simulink model "polyphaseChannelizer"  (R2023b)
settings: Solver=FixedStepDiscrete  StartTime=0.0  StopTime=0.001  RelTol=1e-3
undefined symbols (not defined in the file): parula
libraries: dspobslib x4, dspmlti4 x4, dspmathops x4, radarlib x1, phasedwavlib x1, commdigbbndfm2 x1, commrandsrc3 x1
settings Model: Creator=krsh  LastModifiedBy=krsh
settings SolverCC: AlgebraicLoopSolver=TrustRegion  AutoInsertRateTranBlk=on
settings DataIOCC: LimitDataPoints=on  SaveOutput=off  SignalLogging=off  SaveTime=off
settings OptimizationCC: ReuseModelBlockBuffer=off  LifeSpan=inf  SimCompilerOptimization=on
settings DebuggingCC: AlgebraicLoopMsg=error  SingleTaskRateTransMsg=error  UnconnectedInputMsg=warning  UnconnectedOutputMsg=warning  UnconnectedLineMsg=warning  AllowSymbolicDim=off  SubsystemReferenceDiagnosticForUnitTest=warning  SFUnexpectedBacktrackingDiag=warning  SFNoUnconditionalDefaultTransitionDiag=warning  SFExecutionAtInitializationDiag=none  ArithmeticOperatorsInVariantConditions=warning
settings ModelReferenceCC: EnableRefExpFcnMdlSchedulingChecks=on
settings SFSimCC: SimUseLocalCustomCode=off  CustomCodeUndefinedFunction=UseInterfaceOnly
settings RTWCC: RTWUseLocalCustomCode=off
settings CodeAppCC: StateflowObjectComments=on
settings GRTTargetCC: TargetLangStandard=C89/C90 (ANSI)
settings ConfigComp: CovMetricSettings=dw  CovSaveCumulativeToWorkspaceVar=on  CovSaveSingleToWorkspaceVar=on  CovExternalEMLEnable=off  CovSFcnEnable=off

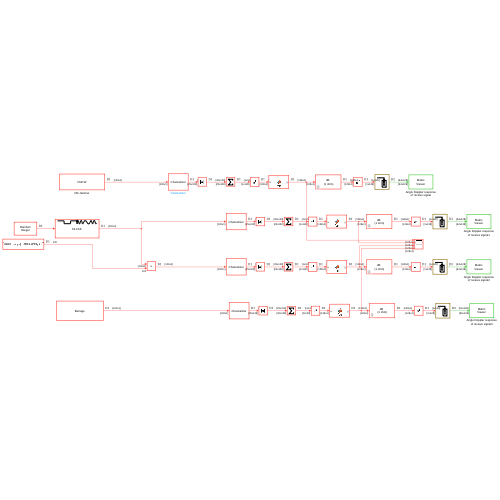
[thumbnail: Simulink's stored preview of the top-level diagram]
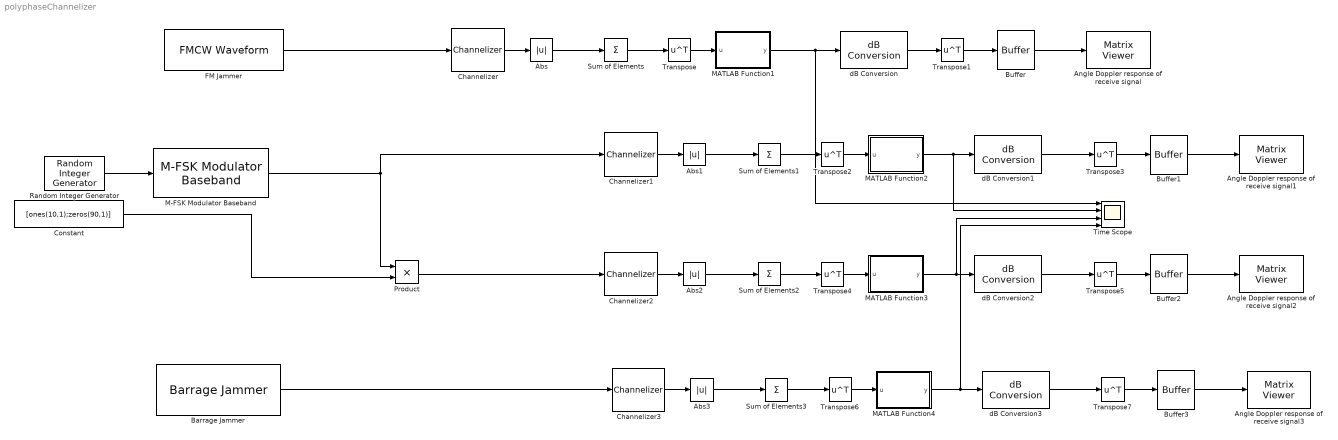
== system polyphaseChannelizer ==
  Abs{,1..3} (4 alike) : Abs  SaturateOnIntegerOverflow=off
  Angle Doppler response of receive signal{,1..3} (4 alike) : dspobslib/Matrix Viewer  ImageParams=off  CMapStr=parula(256)  AxisColorbar=on  AxisParams=off  AxisOrigin=Lower left corner  AxisTickMode=User-defined  XTickRange=[-50e6 50e6]  YTickRange=[0 63]  XLabel=FrequencyBand  YLabel=Sweeps  ZLabel=WaterFallScope  FigPos=[50 360 400 300]  AxisZoom=off
      Angle Doppler response of receive signal settings: YMin=-77.8046  YMax=16.5709
      Angle Doppler response of receive signal1 settings: YMin=-40.3602  YMax=24.0141
      Angle Doppler response of receive signal2 settings: YMin=-34.9744  YMax=8.5209
      Angle Doppler response of receive signal3 settings: YMin=-19.8751  YMax=15.4262
  Barrage Jammer : radarlib/Barrage Jammer  ERP=1  SamplesPerFrameSource=Property  SamplesPerFrame=100  SeedSource=Auto  Seed=0  SimulateUsing=Interpreted execution
  Buffer{,1..3} (4 alike) : Buffer  OutputFrames=off
  Channelizer{,1..3} (4 alike) : dspmlti4/Channelizer  NumFrequencyBands=128  Specification=Number of taps per band and stopband attenuation  DecimationFactor=4  CoefficientsPort=off  NumTapsPerBand=12  StopbandAttenuation=80  LowpassCoefficients=rcosdesign( 0.25, 6, 8, 'sqrt' )  AllowArbitraryInputLength=off  SimulateUsing=Interpreted execution
  Constant : Constant  Value=[ones(10,1);zeros(90,1)]  SampleTime=-1
  FM Jammer : phasedwavlib/FMCW Waveform  SampleRate=100e6  SweepTime=1e-6  SweepBandwidth=30e6  SweepDirection=Triangle  SweepInterval=Symmetric  OutputFormat=Sweeps  NumSamples=100  NumSweeps=1  SimulateUsing=Interpreted execution
  M-FSK Modulator Baseband : commdigbbndfm2/M-FSK Modulator Baseband  M=64  InType=Integer  Enc=Gray  freqSep=100e6/64  phaseType=Continuous  numSamp=100  RateOptions=Enforce single-rate processing  outDataType=double
  MATLAB Function1 : MATLAB Function  TreatAsAtomicUnit=on
  MATLAB Function2 : MATLAB Function  TreatAsAtomicUnit=on
  MATLAB Function3 : MATLAB Function  TreatAsAtomicUnit=on
  MATLAB Function4 : MATLAB Function  TreatAsAtomicUnit=on
  Product : Product
  Random Integer Generator : commrandsrc3/Random Integer Generator  SetSize=64  SeedSource=Auto  Seed=0  SampleTime=1/1e6  SamplesPerFrame=1  OutputDataType=double  SimulateUsing=Interpreted execution
  Sum of Elements{,1..3} (4 alike) : Sum  Inputs=+  CollapseMode=Specified dimension
  Time Scope : Scope  NumInputPorts=4
  Transpose{,1..7} (8 alike) : Math  Operator=transpose
  dB Conversion{,1..3} (4 alike) : dspmathops/dB Conversion  dBtype=dB  intype=Amplitude  R=1  fuzz=off
      settings: LibrarySourceBlock=commutil2/dB Conversion
  wires:
  Random Integer Generator/1 -> M-FSK Modulator Baseband/1
  FM Jammer/1 -> Channelizer/1
  M-FSK Modulator Baseband/1 -> Channelizer1/1, Product/1
  Constant/1 -> Product/2
  Channelizer/1 -> Abs/1
  Abs/1 -> Sum of Elements/1
  Sum of Elements/1 -> Transpose/1
  Transpose/1 -> MATLAB Function1/1(u)
  Transpose1/1 -> Buffer/1
  Buffer/1 -> Angle Doppler response of receive signal/1
  dB Conversion/1 -> Transpose1/1
  dB Conversion1/1 -> Transpose3/1
  Buffer1/1 -> Angle Doppler response of receive signal1/1
  Transpose3/1 -> Buffer1/1
  MATLAB Function2/1(y) -> Time Scope/2, dB Conversion1/1
  Transpose2/1 -> MATLAB Function2/1(u)
  Sum of Elements1/1 -> Transpose2/1
  Abs1/1 -> Sum of Elements1/1
  Channelizer1/1 -> Abs1/1
  Channelizer2/1 -> Abs2/1
  Abs2/1 -> Sum of Elements2/1
  Sum of Elements2/1 -> Transpose4/1
  Transpose4/1 -> MATLAB Function3/1(u)
  MATLAB Function3/1(y) -> Time Scope/3, dB Conversion2/1
  Transpose5/1 -> Buffer2/1
  Buffer2/1 -> Angle Doppler response of receive signal2/1
  dB Conversion2/1 -> Transpose5/1
  Product/1 -> Channelizer2/1
  dB Conversion3/1 -> Transpose7/1
  Buffer3/1 -> Angle Doppler response of receive signal3/1
  Transpose7/1 -> Buffer3/1
  MATLAB Function4/1(y) -> Time Scope/4, dB Conversion3/1
  Transpose6/1 -> MATLAB Function4/1(u)
  Sum of Elements3/1 -> Transpose6/1
  Abs3/1 -> Sum of Elements3/1
  Channelizer3/1 -> Abs3/1
  Barrage Jammer/1 -> Channelizer3/1
  MATLAB Function1/1(y) -> Time Scope/1, dB Conversion/1

== matlab function polyphaseChannelizer/MATLAB Function2 ==
  data: u input; y output
function y = fcn(u)

y = fftshift(u);

== matlab function polyphaseChannelizer/MATLAB Function3 ==
  data: u input; y output
function y = fcn(u)

y = fftshift(u);

== matlab function polyphaseChannelizer/MATLAB Function4 ==
  data: u input; y output
function y = fcn(u)

y = fftshift(u);

== matlab function polyphaseChannelizer/MATLAB Function1 ==
  data: u input; y output
function y = fcn(u)

y = fftshift(u);
